simulink model "observer_model"  (R2018b)
settings: Solver=VariableStepAuto  StartTime=0.0  StopTime=0.5  RelTol=1e-3
values from neighbouring files (symbols this model uses):
  K = 20    [continous_controller.m]    (also in control_input_bound.m = place(sys_discrete.A, sys_discrete.B, discrete_poles); delayed_input.m = place(sys_discrete.A, sys_discrete.B, discrete_poles); discrete_pole_placement.m = place(sys_discrete.A, sys_discrete.B, discrete_poles); pole_placement_delay.m = place(sys.A, sys.B, continous_poles))
  K_obs = K_obs'    [discrete_pole_placement.m]
  k_r = k_r(1)^-1    [discrete_pole_placement.m]    (also in lqr_delay.m = 30)
  sys_discrete = c2d(sys, 2*pi/sampling_freq, 'zoh')    [control_input_bound.m]    (also in delayed_input.m = (c2d(sys, 2*pi/sampling_freq, 'zoh')); discrete_pole_placement.m = (c2d(sys, 2*pi/sampling_freq, 'zoh')); discretization.m; lqr_controller.m)
settings Model: Creator=lorenzoterenzi  LastModifiedBy=lorenzoterenzi

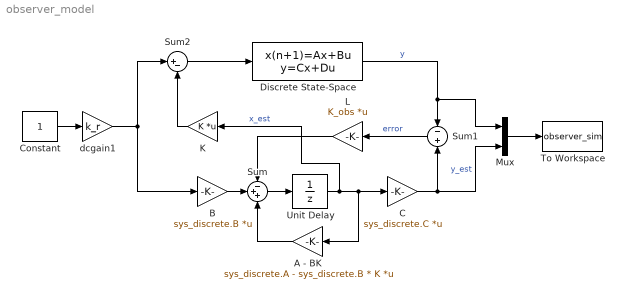
== system observer_model ==
  A - BK : Gain  Gain=sys_discrete.A - sys_discrete.B * K  Multiplication=Matrix(K*u)
  B : Gain  Gain=sys_discrete.B  Multiplication=Matrix(K*u)
  C : Gain  Gain=sys_discrete.C  Multiplication=Matrix(K*u)
  Constant : Constant
  Discrete State-Space : DiscreteStateSpace  A=sys_discrete.A  B=sys_discrete.B  C=sys_discrete.C  D=sys_discrete.D  InitialCondition=[0, 0, 0, 1];  SampleTime=sys_discrete.Ts
  K : Gain  Gain=K  Multiplication=Matrix(K*u)
  L : Gain  Gain=K_obs  Multiplication=Matrix(K*u)
  Mux : Mux  Inputs=2
  Sum : Sum  Inputs=-++
  Sum1 : Sum  Inputs=-|+
  Sum2 : Sum  Inputs=|+-
  To Workspace : ToWorkspace  VariableName=observer_sim  SaveFormat=Timeseries  SampleTime=-1
  Unit Delay : UnitDelay  SampleTime=sys_discrete.Ts
  dcgain1 : Gain  Gain=k_r
  wires:
  Discrete State-Space/1 -> Sum1/1, Mux/1  "y"
  B/1 -> Sum/2
  Unit Delay/1 -> K/1, A - BK/1, C/1  "x_est"
  Sum1/1 -> L/1  "error"
  L/1 -> Sum/1
  Constant/1 -> dcgain1/1
  C/1 -> Sum1/2, Mux/2  "y_est"
  Mux/1 -> To Workspace/1
  A - BK/1 -> Sum/3
  Sum/1 -> Unit Delay/1
  K/1 -> Sum2/2
  dcgain1/1 -> B/1, Sum2/1
  Sum2/1 -> Discrete State-Space/1
